simulink model "Pos_vel_fb"  (R2018a)
settings: Solver=VariableStepAuto  StartTime=0.0  StopTime=40  RelTol=1e-3
settings Model: Creator=thuha  LastModifiedBy=Nguyen Mai

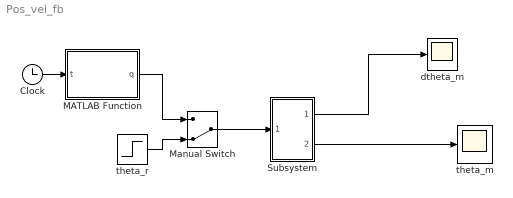
== system Pos_vel_fb ==
  Clock : Clock
      settings: Decimation=40
  MATLAB Function : MATLAB Function  TreatAsAtomicUnit=on
  Manual Switch : ManualSwitch  CurrentSetting=0
  Subsystem : Subsystem
  dtheta_m : Scope
  theta_m : Scope
  theta_r : Step  SampleTime=0
  wires:
  theta_r/1 -> Manual Switch/2
  MATLAB Function/1(q) -> Manual Switch/1
  Clock/1 -> MATLAB Function/1(t)
  Manual Switch/1 -> Subsystem/1(In1)
  Subsystem/1(Out1) -> dtheta_m/1
  Subsystem/2(Out2) -> theta_m/1

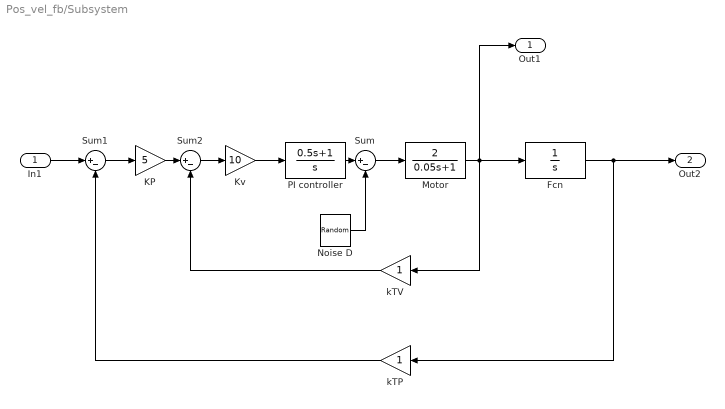
== system Pos_vel_fb/Subsystem ==
  In1 : Inport
  Fcn : TransferFcn  Denominator=[1 0]
  KP : Gain  Gain=5
  Kv : Gain  Gain=10
  Motor : TransferFcn  Numerator=[2]  Denominator=[0.05 1]
  Noise D : UniformRandomNumber  Minimum=-0.01  Maximum=0.01  Seed=24  SampleTime=0.01
  PI controller : TransferFcn  Numerator=[0.5 1]  Denominator=[1 0]
  Sum : Sum  Inputs=|+-
  Sum1 : Sum  Inputs=|+-
  Sum2 : Sum  Inputs=|+-
  kTP : Gain
  kTV : Gain
  Out1 : Outport
  Out2 : Outport  Port=2
  wires:
  Sum/1 -> Motor/1
  Motor/1 -> Out1/1, kTV/1, Fcn/1
  Sum2/1 -> Kv/1
  kTV/1 -> Sum2/2
  Fcn/1 -> Out2/1, kTP/1
  PI controller/1 -> Sum/1
  Noise D/1 -> Sum/2
  Sum1/1 -> KP/1
  kTP/1 -> Sum1/2
  KP/1 -> Sum2/1
  Kv/1 -> PI controller/1
  In1/1 -> Sum1/1

== matlab function Pos_vel_fb/MATLAB Function ==
  data: t input; q output
function q = fcn(t)
t0=0;
tf=40;
tc=4/5;
if t<tc
q=40+(125/8)*t^2;
else
if t<tf-tc
q=30+25*t;
else
q=1020-(125/8)*(40-t)^2;
end
end
